simulink model "command_control_gen"  (R2018b)
settings: Solver=VariableStepAuto  StartTime=0.0  StopTime=10.0  RelTol=1e-3
libraries: SlewAndControlConstrained_Controller_lib x1, PD_Controller_Lib x1, Desaturation_Controller_lib x1
settings Model: Creator=Taylor  LastModifiedBy=Taylor

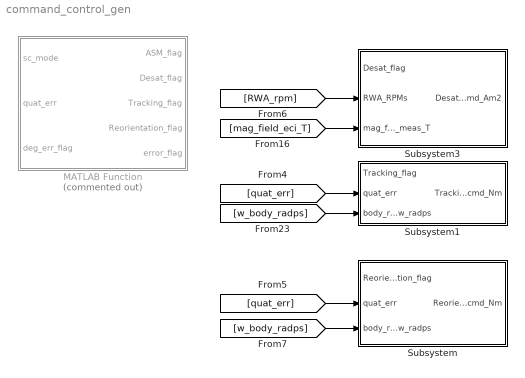
== system command_control_gen ==
  MATLAB Function : MATLAB Function  Commented=on  TreatAsAtomicUnit=on
  Subsystem : Subsystem
  Subsystem1 : Subsystem
  Subsystem3 : Subsystem
  wires:
  [mag_field_eci_T] -> Subsystem3/3(mag_field_vec_meas_T)
  [quat_err] -> Subsystem/2(quat_err)
  [w_body_radps] -> Subsystem/3(body_rates_w_radps)
  [w_body_radps] -> Subsystem1/3(body_rates_w_radps)
  [RWA_rpm] -> Subsystem3/2(RWA_RPMs)
  [quat_err] -> Subsystem1/2(quat_err)

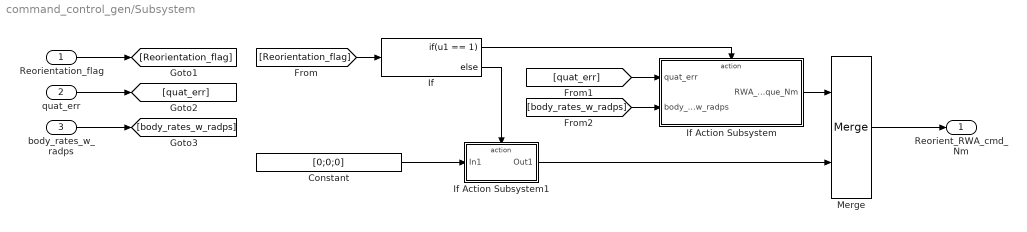
== system command_control_gen/Subsystem ==
  Reorientation_flag : Inport
  quat_err : Inport  Port=2
  body_rates_w_radps : Inport  Port=3
  Constant : Constant  Value=[0;0;0]
  If : If  IfExpression=u1 == 1
  If Action Subsystem : Subsystem  TreatAsAtomicUnit=on
  If Action Subsystem1 : Subsystem  TreatAsAtomicUnit=on
  Merge : Merge
  Reorient_RWA_cmd_Nm : Outport
  wires:
  Merge/1 -> Reorient_RWA_cmd_Nm/1
  If Action Subsystem1/1(Out1) -> Merge/2
  If Action Subsystem/1(RWA_cmd_torque_Nm) -> Merge/1
  If/2 -> If Action Subsystem1/Action
  Constant/1 -> If Action Subsystem1/1(In1)
  If/1 -> If Action Subsystem/Action
  Reorientation_flag/1 -> [Reorientation_flag]
  body_rates_w_radps/1 -> [body_rates_w_radps]
  quat_err/1 -> [quat_err]
  [Reorientation_flag] -> If/1
  [quat_err] -> If Action Subsystem/1(quat_err)
  [body_rates_w_radps] -> If Action Subsystem/2(body_rates_w_radps)

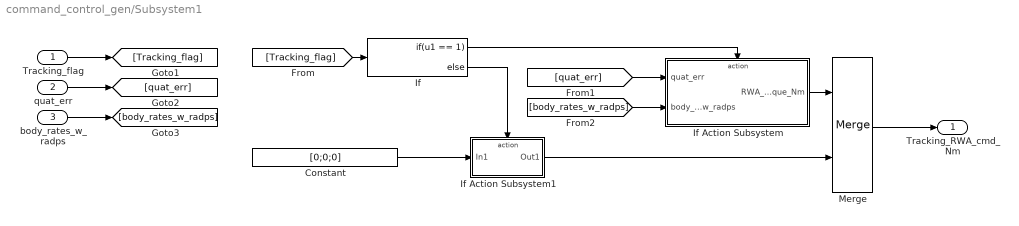
== system command_control_gen/Subsystem1 ==
  Tracking_flag : Inport
  quat_err : Inport  Port=2
  body_rates_w_radps : Inport  Port=3
  Constant : Constant  Value=[0;0;0]
  If : If  IfExpression=u1 == 1
  If Action Subsystem : Subsystem  TreatAsAtomicUnit=on
  If Action Subsystem1 : Subsystem  TreatAsAtomicUnit=on
  Merge : Merge
  Tracking_RWA_cmd_Nm : Outport
  wires:
  Merge/1 -> Tracking_RWA_cmd_Nm/1
  If Action Subsystem1/1(Out1) -> Merge/2
  If Action Subsystem/1(RWA_cmd_torque_Nm) -> Merge/1
  If/2 -> If Action Subsystem1/Action
  Constant/1 -> If Action Subsystem1/1(In1)
  If/1 -> If Action Subsystem/Action
  body_rates_w_radps/1 -> [body_rates_w_radps]
  quat_err/1 -> [quat_err]
  Tracking_flag/1 -> [Tracking_flag]
  [quat_err] -> If Action Subsystem/1(quat_err)
  [body_rates_w_radps] -> If Action Subsystem/2(body_rates_w_radps)
  [Tracking_flag] -> If/1

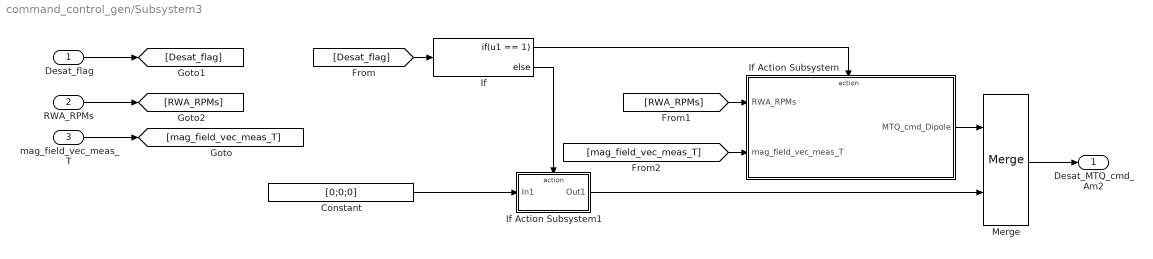
== system command_control_gen/Subsystem3 ==
  Desat_flag : Inport
  RWA_RPMs : Inport  Port=2
  mag_field_vec_meas_T : Inport  Port=3
  Constant : Constant  Value=[0;0;0]
  If : If  IfExpression=u1 == 1
  If Action Subsystem : Subsystem  TreatAsAtomicUnit=on
  If Action Subsystem1 : Subsystem  TreatAsAtomicUnit=on
  Merge : Merge
  Desat_MTQ_cmd_Am2 : Outport
  wires:
  Merge/1 -> Desat_MTQ_cmd_Am2/1
  If Action Subsystem1/1(Out1) -> Merge/2
  If Action Subsystem/1(MTQ_cmd_Dipole) -> Merge/1
  If/2 -> If Action Subsystem1/Action
  Constant/1 -> If Action Subsystem1/1(In1)
  If/1 -> If Action Subsystem/Action
  Desat_flag/1 -> [Desat_flag]
  [Desat_flag] -> If/1
  RWA_RPMs/1 -> [RWA_RPMs]
  mag_field_vec_meas_T/1 -> [mag_field_vec_meas_T]
  [mag_field_vec_meas_T] -> If Action Subsystem/2(mag_field_vec_meas_T)
  [RWA_RPMs] -> If Action Subsystem/1(RWA_RPMs)

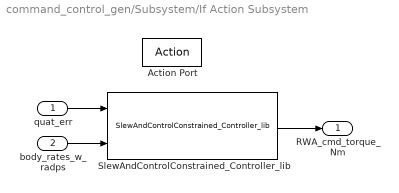
== system command_control_gen/Subsystem/If Action Subsystem ==
  quat_err : Inport
  body_rates_w_radps : Inport  Port=2
  Action Port : ActionPort
  SlewAndControlConstrained_Controller_lib : SlewAndControlConstrained_Controller_lib/SlewAndControlConstrained_Controller_lib  SystemSampleTime=-1
  RWA_cmd_torque_Nm : Outport
  wires:
  quat_err/1 -> SlewAndControlConstrained_Controller_lib/1
  body_rates_w_radps/1 -> SlewAndControlConstrained_Controller_lib/2
  SlewAndControlConstrained_Controller_lib/1 -> RWA_cmd_torque_Nm/1

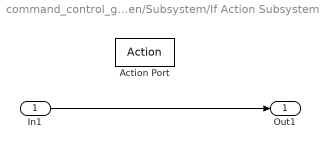
== system command_control_gen/Subsystem/If Action Subsystem1 ==
  In1 : Inport
  Action Port : ActionPort
  Out1 : Outport
  wires:
  In1/1 -> Out1/1

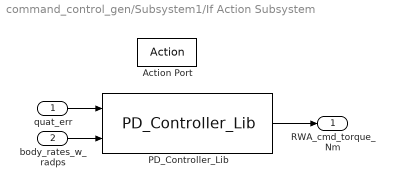
== system command_control_gen/Subsystem1/If Action Subsystem ==
  quat_err : Inport
  body_rates_w_radps : Inport  Port=2
  Action Port : ActionPort
  PD_Controller_Lib : PD_Controller_Lib/PD_Controller_Lib  SystemSampleTime=-1
  RWA_cmd_torque_Nm : Outport
  wires:
  quat_err/1 -> PD_Controller_Lib/1
  body_rates_w_radps/1 -> PD_Controller_Lib/2
  PD_Controller_Lib/1 -> RWA_cmd_torque_Nm/1

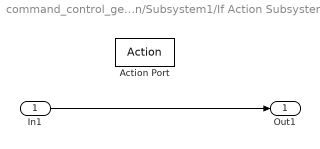
== system command_control_gen/Subsystem1/If Action Subsystem1 ==
  In1 : Inport
  Action Port : ActionPort
  Out1 : Outport
  wires:
  In1/1 -> Out1/1

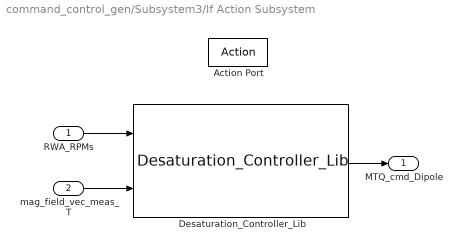
== system command_control_gen/Subsystem3/If Action Subsystem ==
  RWA_RPMs : Inport
  mag_field_vec_meas_T : Inport  Port=2
  Action Port : ActionPort
  Desaturation_Controller_Lib : Desaturation_Controller_lib/Desaturation_Controller_Lib  SystemSampleTime=-1
  MTQ_cmd_Dipole : Outport
  wires:
  RWA_RPMs/1 -> Desaturation_Controller_Lib/1
  Desaturation_Controller_Lib/1 -> MTQ_cmd_Dipole/1
  mag_field_vec_meas_T/1 -> Desaturation_Controller_Lib/2

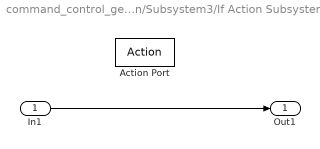
== system command_control_gen/Subsystem3/If Action Subsystem1 ==
  In1 : Inport
  Action Port : ActionPort
  Out1 : Outport
  wires:
  In1/1 -> Out1/1

== matlab function command_control_gen/MATLAB Function ==
  data: sc_mode input; ASM_flag output; quat_err input; Desat_flag output; Tracking_flag output; Reorientation_flag output; error_flag output; deg_err_flag input
% Logic for selecting the gnc control mode. Based on the sc mode, the
% control scheme is selected.
%
% Author: Cole Morgan 11.07.19
%
% 



function [ASM_flag, Desat_flag, Tracking_flag, Reorientation_flag, error_flag]...
                                        = control_selection_logic(sc_mode, quat_err, deg_err_flag)

%#codegen                                    
                                    
%GNC_MODE_LOGIC    GNC sc modes
%
% Chooses controller based on sc mode.
%   mode_logic.low_power        = 1; "safe mode"
%   mode_logic.idle             = 2; "idle/standby mode"
%   mode_logic.stabilize        = 3;
%   mode_logic.nominal          = 4;
%       nominal.desat           = 41;
%       nominal.sun_seek        = 42;
%   mode_logic.point            = 5;
%       point.com               = 51;
%       point.image             = 52;
%       point.exp               = 53;
%
% ----- INPUTS -----
% 
% sc_mode - modes outlined above.
%
% quat_err - error between current and commanded attitude.
%
% ----- OUTPUTS -----
%
% ASM_flag - flag turning Attitude Stabilization (Detumble) controller on/off 
% Desat_flag - flag turning Desaturation controller on/off
% Tracking_flag - flag turning Tracking controller on/off 
% Reorientation_flag - flag turning Large-angle Reorientation controller on/off
% error_flag - indicates this function has failed to find a control scheme
%       when it should have found one.



% Default to no controller selection and some error meaning you didn't ever even trip it.
ASM_flag           = 0;
Desat_flag         = 0;
Tracking_flag      = 0;
Reorientation_flag = 0; 
error_flag         = -1;

% quat_err indicates if large angle reorientation 
% is necessary.
% deg_err is the total error in degrees from the desired
% orientation. If this value is not small, use (or keep using) 
% large-angle reorientation controller until it is small enough to track.
% deg_err = abs(2*acosd(quat_err(1)));

% If sc_mode is not LPM or CLPM
if( sc_mode ~= 1.0 && sc_mode ~= 2.0)
    error_flag = 0;
    
    % engage ASM controller
    if (sc_mode == 3.0)
        ASM_flag = 1;
        
    % engage Desat controller, but Tracking
    % must be maintained.
    elseif (sc_mode == 41.0)
        Desat_flag = 1;
%         Tracking_flag = 1;
        ASM_flag = 1;
        return;
        
    % engage (or keep) Tracking controller engaged in any mode with an  
    % attitude objective. This is the most likely scenario.
    elseif (sc_mode == 42.0 || sc_mode == 51.0 || sc_mode == 52.0 || sc_mode == 53.0)
        Tracking_flag = 1;
        
        % If the angular error is larger than the threshold set in fswParams,
        % (typically less than 3.5 degrees) then a large angle reorientation 
        % is needed.
        if (deg_err_flag) %>= reorientation_controller_threshold)
            Reorientation_flag = 1;
            Tracking_flag = 0;
        end
        
    else
        % indicates we are not in LPM or CLPM and still
        % are not getting a control scheme correctly.
        error_flag = 1;
    end
    
    % Final protection from asking for multiple RWA control schemes.
    % If so, just keep attitude stable.
    check = ASM_flag + Tracking_flag + Reorientation_flag;
    if (check > 1)
        ASM_flag = 1;
        Tracking_flag = 0;
        Reorientation_flag = 0;
        error_flag = 2;
    end
    
    
end
